simulink model "Frequency_Modulation"  (R2025a)
settings: Solver=ode45  StartTime=0.0  StopTime=0.000001  FixedStep=0.000000001  RelTol=1e-3
settings Model: Creator=anunn  LastModifiedBy=anunn

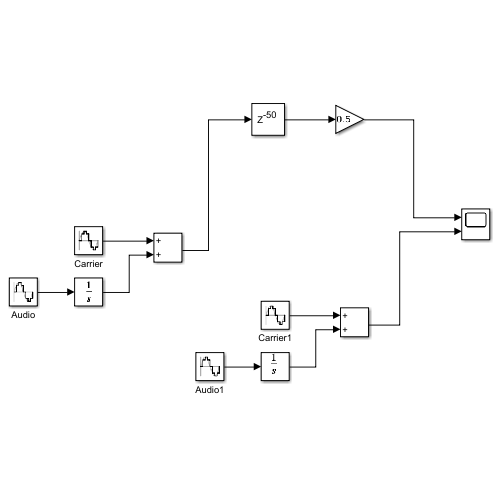
[thumbnail: Simulink's stored preview of the top-level diagram]
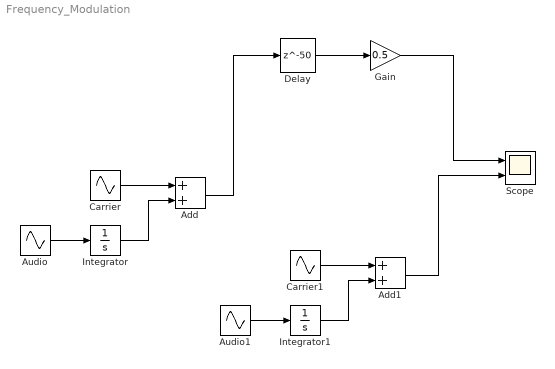
== system Frequency_Modulation ==
  Add : Sum
  Add1 : Sum
  Audio : Sin  Frequency=6283185.3071796  SampleTime=0.000000001
  Audio1 : Sin  Frequency=6283185.3071796  SampleTime=0.000000001
  Carrier : Sin  Frequency=628318530.71796  SampleTime=0.000000001
  Carrier1 : Sin  Frequency=628318530.71796  SampleTime=0.000000001
  Delay : Delay  DelayLength=50
  Gain : Gain  Gain=0.5
  Integrator : Integrator
  Integrator1 : Integrator
  Scope : Scope  NumInputPorts=2
      settings: ActiveDisplayYMinimum=-6.1595541757450842  ActiveDisplayYMaximum=5.9494227335995475
  wires:
  Carrier/1 -> Add/1
  Delay/1 -> Gain/1
  Gain/1 -> Scope/1
  Audio/1 -> Integrator/1
  Add/1 -> Delay/1
  Integrator/1 -> Add/2
  Add1/1 -> Scope/2
  Audio1/1 -> Integrator1/1
  Carrier1/1 -> Add1/1
  Integrator1/1 -> Add1/2
